simulink model "ansiOctComp"  (R2018a)
settings: Solver=VariableStepAuto  StartTime=0.0  StopTime=0.001  RelTol=1e-3
undefined symbols (not defined in the file): fdesignblkfcn, G1, G2, G3, G4, G5, G6, G7, G8, gcbh, get, T
libraries: dspsrcs4 x1, dspxfrm3 x1, dspobslib x1
(part 2 of 3)

== system ansiOctComp/Filter Bank /Filter 7/Bandpass Filter ==
  In : Inport
  Generated Filter Block : DiscreteFir  Tag=BlockMethodSubSystem  Coefficients=[0.000688747021894905889 2.18684298008015856e-05 -0.000747774121627521084 -0.000944058309513606591 -0.0003253492168160309 9.23101405120965485e-05 -0.000131668261710039206 0.000278299081757325871 0.00203685546617077794 0.00282127501297776626 -0.000224709806789325146 -0.00520584422999511177 -0.00594883627287124024 0.000104776300548475431 0.00699311488289822321 0.00678303313259411272 -0.000102973163323512827 -0.00534202521083943123 -0.00384222786058355031 0.000225635118397079837 0.000786570913460919751 -0.00113558835506687812 -0.000356549883511292831 0.00316551500606420452 0.00402210419483252021 0.000322671204025696797 -0.00302827437643997388 -0.00216241189084108009 -0.000100813788313752328 -0.000946319429482982534 -0.00249356303439283132 -0.000132893301647272187 0.00440682241811530574 0.00478680562478373157 0.000166602611108409172 -0.00313585876482802518 -0.00167151510761213767 1.82691025068816831e-05 -0.0021013983861952008 -0.00395901110293506858 -0.000207114547394701611 0.00567024530585669498 0.00573968097265152143 0.000174823472250806768 -0.00296323872407792347 -0.000848885771231672344 6.02451606138625724e-05 -0.00386543105769642436 -0.00596799938366046438 -0.000241959352823016387 0.00725476107922014279 0.00675905125520697651 0.000156525444502864661 -0.00239642366385430005 0.000584860770044941854 0.000116746090016668636 -0.00637431642816130468 -0.00864825281754785444 -0.000274770149259543229 0.00906406170058568321 0.00767549981510917429 0.000128325194659888349 -0.00109798340411188574 0.00298635822444113554 0.000172013986760184787 -0.00995471786868828978 -0.0122262860177205709 -0.000289429179599843146 0.0110718951047434951 0.00828444979299942583 8.00096111541152974e-05 0.00143940511550613237 0.0069799678032253917 0.000230656445653469946 -0.0152584825098764434 -0.0172511918860694773 -0.000290673659826494631 0.0133414677838347932 0.00830270700510185242 2.19011819696309385e-05 0.00630234256282785968 0.0139879881369137093 0.000280183979399447648 -0.0240273714837147996 -0.0252923712533665752 -0.000272683548033014929 0.0162592575259398707 0.00706560096826768826 -4.35748078964608848e-05 0.0169311165912110519 0.0289161122637894945 0.000315185308307668402 -0.0431671491461131721 -0.0431328019381585631 -0.000233050029664418762 0.0220958062178700232 0.00150542181965559411 -0.000114144512323115406 0.0556632812146515277 0.0889235674356774614 0.000335148073650662348 -0.151569396799215494 -0.17692677818321656 -0.000178950765438543047 0.204075838377702878 0.204075838377702878 -0.000178950765438543047 -0.17692677818321656 -0.151569396799215494 0.000335148073650662348 0.0889235674356774614 0.0556632812146515277 -0.000114144512323115406 0.00150542181965559411 0.0220958062178700232 -0.000233050029664418762 -0.0431328019381585631 -0.0431671491461131721 0.000315185308307668402 0.0289161122637894945 0.0169311165912110519 -4.35748078964608848e-05 0.00706560096826768826 0.0162592575259398707 -0.000272683548033014929 -0.0252923712533665752 -0.0240273714837147996 0.000280183979399447648 0.0139879881369137093 0.00630234256282785968 2.19011819696309385e-05 0.00830270700510185242 0.0133414677838347932 -0.000290673659826494631 -0.0172511918860694773 -0.0152584825098764434 0.000230656445653469946 0.0069799678032253917 0.00143940511550613237 8.00096111541152974e-05 0.00828444979299942583 0.0110718951047434951 -0.000289429179599843146 -0.0122262860177205709 -0.00995471786868828978 0.000172013986760184787 0.00298635822444113554 -0.00109798340411188574 0.000128325194659888349 0.00767549981510917429 0.00906406170058568321 -0.000274770149259543229 -0.00864825281754785444 -0.00637431642816130468 0.000116746090016668636 0.000584860770044941854 -0.00239642366385430005 0.000156525444502864661 0.00675905125520697651 0.00725476107922014279 -0.000241959352823016387 -0.00596799938366046438 -0.00386543105769642436 6.02451606138625724e-05 -0.000848885771231672344 -0.00296323872407792347 0.000174823472250806768 0.00573968097265152143 0.00567024530585669498 ...(+984 chars)]  InputProcessing=Columns as channels (frame based)
  Out : Outport
  wires:
  In/1 -> Generated Filter Block/1
  Generated Filter Block/1 -> Out/1

== system ansiOctComp/Filter Bank /Filter 8/Bandpass Filter ==
  In : Inport
  Generated Filter Block : DiscreteFir  Tag=BlockMethodSubSystem  Coefficients=[0.00208920521587915246 -0.00239512818882031209 -0.00053855600712965075 0.00150475259248641934 0.00252544250182454386 -0.00262685013507397373 -0.00682438869370431342 0.0130444383713146095 -0.00467990488077754934 -0.00666027455039981762 0.0065164932128488522 -0.001729553695465373 0.0027950984838265476 -0.00392121882782151248 0.000137629180377313461 0.000691755262694491112 0.00294733775033876894 -0.00196841445717181639 -0.00248992082802597988 0.0017519958426288815 0.00046966668933724748 0.00262630220439261791 -0.00459492818474551735 0.00106769995546806499 -0.000389444490693690399 0.0038542944042112481 -0.00236351548851125191 -0.00188112642215912135 0.000257224238094455951 0.00169589471518602508 0.00265878035526694121 -0.00473885524561892639 0.000805894918949866213 -0.00119578655816939298 0.00565818675776582573 -0.00335162697798689103 -0.00121382357210092972 -0.00163666245933176305 0.0034257953253684398 0.00255966812741642222 -0.00452860735243412835 -0.000172673285062963013 -0.00174515950402045128 0.00762753758969023869 -0.00427652780988023798 -0.000415142871464710037 -0.00434745674088348692 0.00594572238940444236 0.00198782770890439412 -0.00339539960772064281 -0.00235619635441489984 -0.00174154397900754031 0.00932818297228426609 -0.00456412086188246781 0.000211468997190310308 -0.00783040750598629036 0.00912027015947805379 0.00101066349951296286 -0.000993201992272878427 -0.00621406621928159274 -0.000933278796841543546 0.010374879780530635 -0.0035058074009965837 0.000183774544916749492 -0.0119932781167965165 0.0127164419702139927 -0.000118627653125519638 0.00306665921662160369 -0.0124560410028310802 0.00103531382505865003 0.0102247032262783432 0.000114107468776567908 -0.00138498443566570872 -0.0167418874624110751 0.0162963794100802369 -0.000676383865222395376 0.00932848769675900108 -0.0223771025899010684 0.0044915073428323047 0.00831785564204764148 0.00860697865906221923 -0.00610825532917689748 -0.0226525365322748432 0.0193817763974839519 0.00104923132526923502 0.0197960166547991728 -0.0404947799116348456 0.0104095040355148393 0.00325393347708273582 0.0303041591252078656 -0.019893795865867276 -0.0338370562033461705 0.021461701983966644 0.0127466721478665217 0.0484039343744557954 -0.100143205815215075 0.0276522419142769607 -0.0181644642821803294 0.171371970609715235 -0.150178366693390353 -0.218300812871885463 0.466638075069337244 -0.218300812871885463 -0.150178366693390353 0.171371970609715235 -0.0181644642821803294 0.0276522419142769607 -0.100143205815215075 0.0484039343744557954 0.0127466721478665217 0.021461701983966644 -0.0338370562033461705 -0.019893795865867276 0.0303041591252078656 0.00325393347708273582 0.0104095040355148393 -0.0404947799116348456 0.0197960166547991728 0.00104923132526923502 0.0193817763974839519 -0.0226525365322748432 -0.00610825532917689748 0.00860697865906221923 0.00831785564204764148 0.0044915073428323047 -0.0223771025899010684 0.00932848769675900108 -0.000676383865222395376 0.0162963794100802369 -0.0167418874624110751 -0.00138498443566570872 0.000114107468776567908 0.0102247032262783432 0.00103531382505865003 -0.0124560410028310802 0.00306665921662160369 -0.000118627653125519638 0.0127164419702139927 -0.0119932781167965165 0.000183774544916749492 -0.0035058074009965837 0.010374879780530635 -0.000933278796841543546 -0.00621406621928159274 -0.000993201992272878427 0.00101066349951296286 0.00912027015947805379 -0.00783040750598629036 0.000211468997190310308 -0.00456412086188246781 0.00932818297228426609 -0.00174154397900754031 -0.00235619635441489984 -0.00339539960772064281 0.00198782770890439412 0.00594572238940444236 -0.00434745674088348692 -0.000415142871464710037 -0.00427652780988023798 0.00762753758969023869 -0.00174515950402045128 -0.000172673285062963013 -0.00452860735243412835 0.00255966812741642222 0.0034257953253684398 -0.00163666245933176305 -0.00121382357210092972 -0.00335162697798689103 0.00565818675776582573 -0.00119578655816939298 0.000805894918949866213 -0.00473885524561892639 ...(+724 chars)]  InputProcessing=Columns as channels (frame based)
  Out : Outport
  wires:
  In/1 -> Generated Filter Block/1
  Generated Filter Block/1 -> Out/1
